simulink model "testingsecondcontroller"  (R2021b)
settings: Solver=VariableStepAuto  StartTime=0.0  StopTime=10.0  RelTol=1e-3
settings Model: Creator=Asus  LastModifiedBy=Matina Kaviani
settings SolverCC: AlgebraicLoopSolver=TrustRegion
settings DebuggingCC: SFMachineParentedDataDiag=warning

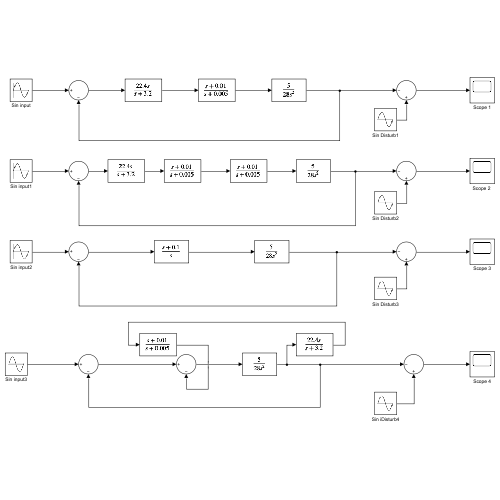
[thumbnail: Simulink's stored preview of the top-level diagram]
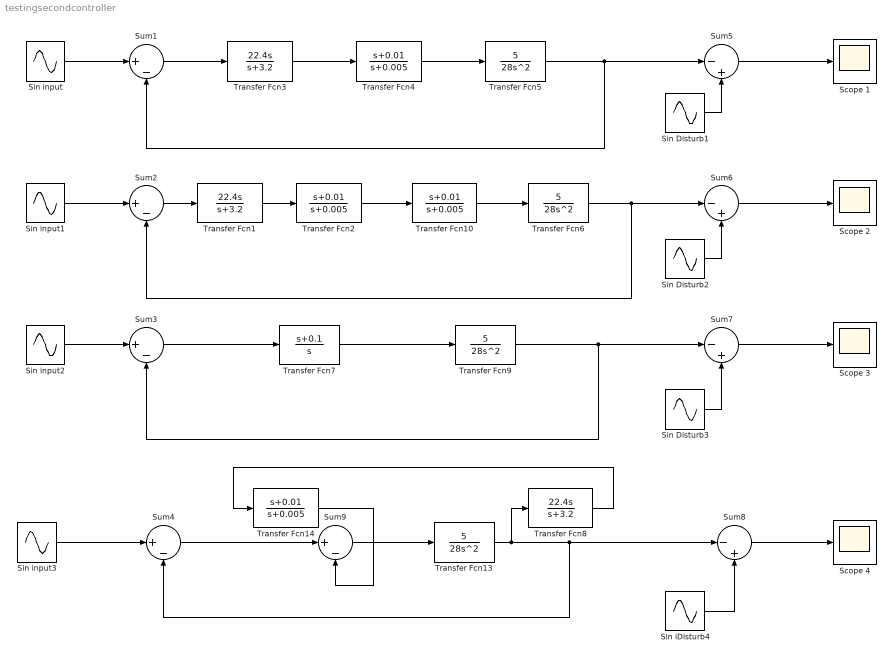
== system testingsecondcontroller ==
  Scope 1 : Scope
  "Scope 2 " : Scope
  Scope 3 : Scope
  Scope 4 : Scope
  Sin Disturb1 : Sin  Frequency=2*pi  SampleTime=0
  Sin Disturb2 : Sin  Frequency=2*pi  SampleTime=0
  Sin Disturb3 : Sin  Frequency=2*pi  SampleTime=0
  Sin iDisturb4 : Sin  Frequency=2*pi  SampleTime=0
  Sin input{,1..3} (4 alike) : Sin  Frequency=2*pi  SampleTime=0
  Sum{1..4,9} (5 alike) : Sum  Inputs=|+-
  Sum{5..8} (4 alike) : Sum  Inputs=|-+
  Transfer Fcn1 : TransferFcn  Numerator=[22.4 0]  Denominator=[1 3.2]
  Transfer Fcn{2,4,10,14} (4 alike) : TransferFcn  Numerator=[1 0.01]  Denominator=[1 0.005]
  Transfer Fcn{5..6,9,13} (4 alike) : TransferFcn  Numerator=[0 5]  Denominator=[28 0 0]
  Transfer Fcn3 : TransferFcn  Numerator=[22.4 0]  Denominator=[1 3.2]
  Transfer Fcn7 : TransferFcn  Numerator=[1 0.1]  Denominator=[1 0]
  Transfer Fcn8 : TransferFcn  Numerator=[22.4 0]  Denominator=[1 3.2]
  wires:
  Transfer Fcn3/1 -> Transfer Fcn4/1
  Sin input/1 -> Sum1/1
  Sum1/1 -> Transfer Fcn3/1
  Transfer Fcn4/1 -> Transfer Fcn5/1
  Sin input1/1 -> Sum2/1
  Sum2/1 -> Transfer Fcn1/1
  Transfer Fcn6/1 -> Sum2/2, Sum6/1
  Transfer Fcn1/1 -> Transfer Fcn2/1
  Sin input2/1 -> Sum3/1
  Transfer Fcn9/1 -> Sum3/2, Sum7/1
  Transfer Fcn2/1 -> Transfer Fcn10/1
  Transfer Fcn10/1 -> Transfer Fcn6/1
  Transfer Fcn13/1 -> Sum4/2, Sum8/1, Transfer Fcn8/1
  Sin input3/1 -> Sum4/1
  Sum3/1 -> Transfer Fcn7/1
  Transfer Fcn7/1 -> Transfer Fcn9/1
  Transfer Fcn5/1 -> Sum5/1, Sum1/2
  Sin Disturb1/1 -> Sum5/2
  Sum5/1 -> Scope 1/1
  Sum6/1 -> "Scope 2 "/1
  Sin Disturb2/1 -> Sum6/2
  Sum7/1 -> Scope 3/1
  Sin Disturb3/1 -> Sum7/2
  Sum8/1 -> Scope 4/1
  Sin iDisturb4/1 -> Sum8/2
  Sum9/1 -> Transfer Fcn13/1
  Transfer Fcn8/1 -> Transfer Fcn14/1
  Transfer Fcn14/1 -> Sum9/2
  Sum4/1 -> Sum9/1
